simulink model "AirCtl_Mon"  (R2016b)
settings: configuration reference "CodeGenConfigSet" (kept outside this file)
values from neighbouring files (symbols this model uses):
  AirCtl_dnEngTrans_C = Calibration.Parameter    [init_AirCtl_Mon.m]    (also in init_AirCtl_Mon_SIL.m = Simulink.Parameter)
  AirCtl_dqLeadTrans_C = Calibration.Parameter    [init_AirCtl_Mon.m]    (also in init_AirCtl_Mon_SIL.m = Simulink.Parameter)
  AirCtl_drAPPTrans_C = Calibration.Parameter    [init_AirCtl_Mon.m]    (also in init_AirCtl_Mon_SIL.m = Simulink.Parameter)
  AirCtl_facActDesVal_C = Calibration.Parameter    [init_AirCtl_Mon.m]    (also in init_AirCtl_Mon_SIL.m = Simulink.Parameter)
  AirCtl_facEngTempSmkHysCor_CUR = Calibration.Parameter    [init_AirCtl_Mon.m]    (also in init_AirCtl_Mon_SIL.m = Simulink.Parameter)
  AirCtl_facEngTempSmkHysCor_CURX = Calibration.Parameter    [init_AirCtl_Mon.m]    (also in init_AirCtl_Mon_SIL.m = Simulink.Parameter)
  AirCtl_facEnvPresSmkHysCor_CUR = Calibration.Parameter    [init_AirCtl_Mon.m]    (also in init_AirCtl_Mon_SIL.m = Simulink.Parameter)
  AirCtl_facEnvPresSmkHysCor_CURX = Calibration.Parameter    [init_AirCtl_Mon.m]    (also in init_AirCtl_Mon_SIL.m = Simulink.Parameter)
  AirCtl_mMaxDvt_MAP = Calibration.Parameter    [init_AirCtl_Mon.m]    (also in init_AirCtl_Mon_SIL.m = Simulink.Parameter)
  AirCtl_mMaxDvt_MAPX = Calibration.Parameter    [init_AirCtl_Mon.m]    (also in init_AirCtl_Mon_SIL.m = Simulink.Parameter)
  AirCtl_mMaxDvt_MAPY = Calibration.Parameter    [init_AirCtl_Mon.m]    (also in init_AirCtl_Mon_SIL.m = Simulink.Parameter)
  AirCtl_mMinDvt_MAP = Calibration.Parameter    [init_AirCtl_Mon.m]    (also in init_AirCtl_Mon_SIL.m = Simulink.Parameter)
  AirCtl_mMinDvt_MAPX = Calibration.Parameter    [init_AirCtl_Mon.m]    (also in init_AirCtl_Mon_SIL.m = Simulink.Parameter)
  AirCtl_mMinDvt_MAPY = Calibration.Parameter    [init_AirCtl_Mon.m]    (also in init_AirCtl_Mon_SIL.m = Simulink.Parameter)
  AirCtl_nLoIdl_C = Calibration.Parameter    [init_AirCtl_Mon.m]    (also in init_AirCtl_Mon_SIL.m = Simulink.Parameter)
  AirCtl_nOvrRun_C = Calibration.Parameter    [init_AirCtl_Mon.m]    (also in init_AirCtl_Mon_SIL.m = Simulink.Parameter)
  AirCtl_numAirTempMon_C = Calibration.Parameter    [init_AirCtl_Mon.m]    (also in init_AirCtl_Mon_SIL.m = Simulink.Parameter)
  AirCtl_numEngTempMon_C = Calibration.Parameter    [init_AirCtl_Mon.m]    (also in init_AirCtl_Mon_SIL.m = Simulink.Parameter)
  AirCtl_pAirHi_C = Calibration.Parameter    [init_AirCtl_Mon.m]    (also in init_AirCtl_Mon_SIL.m = Simulink.Parameter)
  AirCtl_pAirLo_C = Calibration.Parameter    [init_AirCtl_Mon.m]    (also in init_AirCtl_Mon_SIL.m = Simulink.Parameter)
  AirCtl_qEngTempSmkHysCor_MAP = Calibration.Parameter    [init_AirCtl_Mon.m]    (also in init_AirCtl_Mon_SIL.m = Simulink.Parameter)
  AirCtl_qEngTempSmkHysCor_MAPX = Calibration.Parameter    [init_AirCtl_Mon.m]    (also in init_AirCtl_Mon_SIL.m = Simulink.Parameter)
  AirCtl_qEngTempSmkHysCor_MAPY = Calibration.Parameter    [init_AirCtl_Mon.m]    (also in init_AirCtl_Mon_SIL.m = Simulink.Parameter)
  AirCtl_qEnvPresSmkHysCor_MAP = Calibration.Parameter    [init_AirCtl_Mon.m]    (also in init_AirCtl_Mon_SIL.m = Simulink.Parameter)
  AirCtl_qEnvPresSmkHysCor_MAPX = Calibration.Parameter    [init_AirCtl_Mon.m]    (also in init_AirCtl_Mon_SIL.m = Simulink.Parameter)
  AirCtl_qEnvPresSmkHysCor_MAPY = Calibration.Parameter    [init_AirCtl_Mon.m]    (also in init_AirCtl_Mon_SIL.m = Simulink.Parameter)
  AirCtl_qOvrRun_C = Calibration.Parameter    [init_AirCtl_Mon.m]    (also in init_AirCtl_Mon_SIL.m = Simulink.Parameter)
  AirCtl_qSmkHys_MAP = Calibration.Parameter    [init_AirCtl_Mon.m]    (also in init_AirCtl_Mon_SIL.m = Simulink.Parameter)
  AirCtl_qSmkHys_MAPX = Calibration.Parameter    [init_AirCtl_Mon.m]    (also in init_AirCtl_Mon_SIL.m = Simulink.Parameter)
  AirCtl_qSmkHys_MAPY = Calibration.Parameter    [init_AirCtl_Mon.m]    (also in init_AirCtl_Mon_SIL.m = Simulink.Parameter)
  AirCtl_qSwtSmkHi_C = Calibration.Parameter    [init_AirCtl_Mon.m]    (also in init_AirCtl_Mon_SIL.m = Simulink.Parameter)
  AirCtl_qSwtSmkLo_C = Calibration.Parameter    [init_AirCtl_Mon.m]    (also in init_AirCtl_Mon_SIL.m = Simulink.Parameter)
  AirCtl_rEGRDflVal_CA = Calibration.Parameter    [init_AirCtl_Mon.m]    (also in init_AirCtl_Mon_SIL.m = Simulink.Parameter)
  AirCtl_rTVADflVal_CA = Calibration.Parameter    [init_AirCtl_Mon.m]    (also in init_AirCtl_Mon_SIL.m = Simulink.Parameter)
  AirCtl_stPrioMon_CA = Calibration.Parameter    [init_AirCtl_Mon.m]    (also in init_AirCtl_Mon_SIL.m = Simulink.Parameter)
  AirCtl_swtGovDvtMonEna_C = Calibration.Parameter    [init_AirCtl_Mon.m]    (also in init_AirCtl_Mon_SIL.m = Simulink.Parameter)
  AirCtl_tAirCldHi_C = Calibration.Parameter    [init_AirCtl_Mon.m]    (also in init_AirCtl_Mon_SIL.m = Simulink.Parameter)
  AirCtl_tAirCldLo_C = Calibration.Parameter    [init_AirCtl_Mon.m]    (also in init_AirCtl_Mon_SIL.m = Simulink.Parameter)
  AirCtl_tAirWrmHi_C = Calibration.Parameter    [init_AirCtl_Mon.m]    (also in init_AirCtl_Mon_SIL.m = Simulink.Parameter)
  AirCtl_tAirWrmLo_C = Calibration.Parameter    [init_AirCtl_Mon.m]    (also in init_AirCtl_Mon_SIL.m = Simulink.Parameter)
  AirCtl_tClntCldHi_C = Calibration.Parameter    [init_AirCtl_Mon.m]    (also in init_AirCtl_Mon_SIL.m = Simulink.Parameter)
  AirCtl_tClntCldLo_C = Calibration.Parameter    [init_AirCtl_Mon.m]    (also in init_AirCtl_Mon_SIL.m = Simulink.Parameter)
  AirCtl_tClntWrmHi_C = Calibration.Parameter    [init_AirCtl_Mon.m]    (also in init_AirCtl_Mon_SIL.m = Simulink.Parameter)
  AirCtl_tClntWrmLo_C = Calibration.Parameter    [init_AirCtl_Mon.m]    (also in init_AirCtl_Mon_SIL.m = Simulink.Parameter)
  AirCtl_tiCldStrt_CUR = Calibration.Parameter    [init_AirCtl_Mon.m]    (also in init_AirCtl_Mon_SIL.m = Simulink.Parameter)
  AirCtl_tiCldStrt_CURX = Calibration.Parameter    [init_AirCtl_Mon.m]    (also in init_AirCtl_Mon_SIL.m = Simulink.Parameter)
  AirCtl_tiClth_C = Calibration.Parameter    [init_AirCtl_Mon.m]    (also in init_AirCtl_Mon_SIL.m = Simulink.Parameter)
  AirCtl_tiDynSmkDly_C = Calibration.Parameter    [init_AirCtl_Mon.m]    (also in init_AirCtl_Mon_SIL.m = Simulink.Parameter)
  AirCtl_tiGovDvtMaxDebDef_C = Calibration.Parameter    [init_AirCtl_Mon.m]    (also in init_AirCtl_Mon_SIL.m = Simulink.Parameter)
  AirCtl_tiGovDvtMaxDebOk_C = Calibration.Parameter    [init_AirCtl_Mon.m]    (also in init_AirCtl_Mon_SIL.m = Simulink.Parameter)
  AirCtl_tiGovDvtMinDebDef_C = Calibration.Parameter    [init_AirCtl_Mon.m]    (also in init_AirCtl_Mon_SIL.m = Simulink.Parameter)
  AirCtl_tiGovDvtMinDebOk_C = Calibration.Parameter    [init_AirCtl_Mon.m]    (also in init_AirCtl_Mon_SIL.m = Simulink.Parameter)
  AirCtl_tiLoIdl_C = Calibration.Parameter    [init_AirCtl_Mon.m]    (also in init_AirCtl_Mon_SIL.m = Simulink.Parameter)
  AirCtl_tiStatSmkDly_C = Calibration.Parameter    [init_AirCtl_Mon.m]    (also in init_AirCtl_Mon_SIL.m = Simulink.Parameter)
  AirCtl_tiTransDly_C = Calibration.Parameter    [init_AirCtl_Mon.m]    (also in init_AirCtl_Mon_SIL.m = Simulink.Parameter)
  AirCtl_uBattThres_C = Calibration.Parameter    [init_AirCtl_Mon.m]    (also in init_AirCtl_Mon_SIL.m = Simulink.Parameter)
  ASMod_numBnk_C = Calibration.Parameter    [init_AirCtl_Mon.m]    (also in init_AirCtl_Mon_SIL.m = Simulink.Parameter)
  Epm_numCyl_C = Calibration.Parameter    [init_AirCtl_Mon.m]    (also in init_AirCtl_Mon_SIL.m = Simulink.Parameter)
undefined symbols (not defined in the file or in its folder): AirCtl_Mon_DT, EngState_conv, Switch_conv
libraries: simulink x45, CXLib x23
(part 2 of 4)

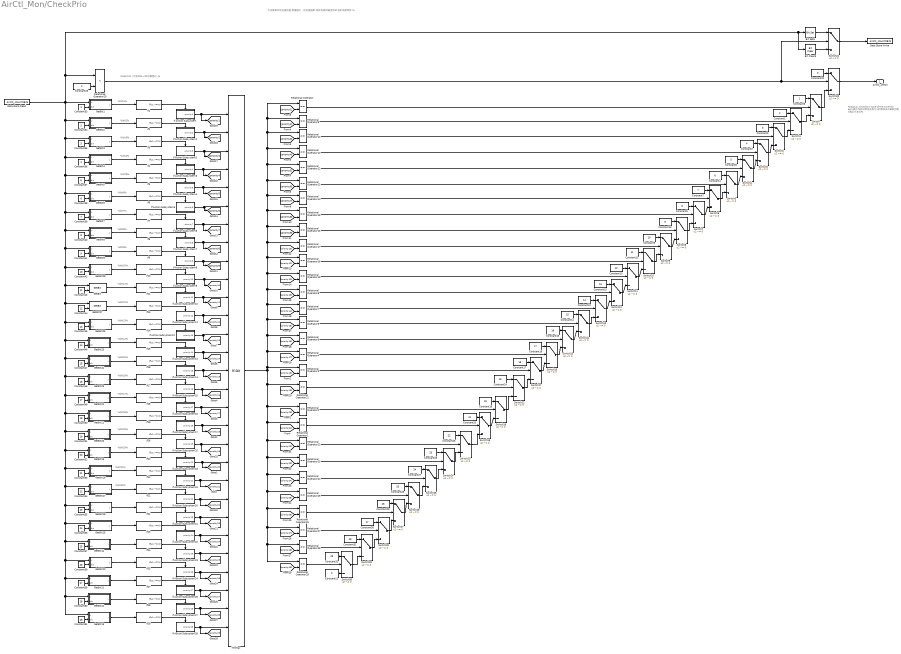
== system AirCtl_Mon/CheckPrio ==
  note: %bit19%
  note: %bit22%
  note: %bit21%
  note: %bit20%
  note: %bit18%
  note: %bit17%
  note: %bit16%
  note: %bit15%
  note: %bit14%
  note: %bit13%
  note: %bit12%
  note: %bit11%
  note: %bit10%
  note: %bit9%
  note: %bit8%
  note: %bit7%
  note: %bit6%
  note: %bit5%
  note: %bit4%
  note: %bit3%
  note: %关断条件优先级检查
      | 数值越大，优先级越高,同优先级时输出低bit位的关断条件 %
  note: %Status: shutdown case of the governor
      | eg:1表示当前中断优先级为1的请求关闭EGR控制
      | 0表示不关闭%
  note: %bit1%
  note: %bit2%
  note: %Normal（所有bit1~31位都是0）%
  Bit Clear5 : simulink/Logic and Bit Operations/Bit Clear  iBit=0
  Bit Set5 : simulink/Logic and Bit Operations/Bit Set  iBit=0
  Constant1 : Constant  Value=2  OutDataTypeStr=Inherit: Inherit via back propagation
  Constant10 : Constant  Value=12  OutDataTypeStr=Inherit: Inherit via back propagation
  Constant11 : Constant  Value=11  OutDataTypeStr=Inherit: Inherit via back propagation
  Constant12 : Constant  Value=14  OutDataTypeStr=Inherit: Inherit via back propagation
  Constant13 : Constant  Value=9  OutDataTypeStr=Inherit: Inherit via back propagation
  Constant14 : Constant  Value=15  OutDataTypeStr=Inherit: Inherit via back propagation
  Constant15 : Constant  Value=13  OutDataTypeStr=Inherit: Inherit via back propagation
  Constant16 : Constant  Value=16  OutDataTypeStr=Inherit: Inherit via back propagation
  Constant17 : Constant  Value=18  OutDataTypeStr=Inherit: Inherit via back propagation
  Constant18 : Constant  Value=20  OutDataTypeStr=Inherit: Inherit via back propagation
  Constant19 : Constant  Value=17  OutDataTypeStr=Inherit: Inherit via back propagation
  Constant2 : Constant  Value=4  OutDataTypeStr=Inherit: Inherit via back propagation
  Constant20 : Constant  Value=21  OutDataTypeStr=Inherit: Inherit via back propagation
  Constant21 : Constant  Value=0  OutDataTypeStr=Inherit: Inherit via back propagation
  Constant22 : Constant  Value=0  OutDataTypeStr=Inherit: Inherit via back propagation
  Constant23 : Constant  RequirementInfo={'other' 'APP_requirements.doc' '@Simulink_requirement_item_25' 'true' '手动开关' '' } %GIDa_9ff8e7a4_19db_42e9_b888_d3f27c0a2a42  Value=2  OutDataTypeStr=Inherit: Inherit via back propagation
  Constant24 : Constant  Value=19  OutDataTypeStr=Inherit: Inherit via back propagation
  Constant25 : Constant  Value=22  OutDataTypeStr=Inherit: Inherit via back propagation
  Constant26 : Constant  Value=23  OutDataTypeStr=Inherit: Inherit via back propagation
  Constant27 : Constant  Value=24  OutDataTypeStr=Inherit: Inherit via back propagation
  Constant28 : Constant  Value=25  OutDataTypeStr=Inherit: Inherit via back propagation
  Constant29 : Constant  Value=26  OutDataTypeStr=Inherit: Inherit via back propagation
  Constant3 : Constant  Value=3  OutDataTypeStr=Inherit: Inherit via back propagation
  Constant30 : Constant  Value=27  OutDataTypeStr=Inherit: Inherit via back propagation
  Constant31 : Constant  Value=28  OutDataTypeStr=Inherit: Inherit via back propagation
  Constant32 : Constant  Value=29  OutDataTypeStr=Inherit: Inherit via back propagation
  Constant33 : Constant  RequirementInfo={'other' 'APP_requirements.doc' '@Simulink_requirement_item_25' 'true' '手动开关' '' } %GIDa_8dd0c6e6_ea60_49d7_b46b_ab438e246230  OutDataTypeStr=uint8
  Constant34 : Constant  RequirementInfo={'other' 'APP_requirements.doc' '@Simulink_requirement_item_25' 'true' '手动开关' '' } %GIDa_459ecf2d_1b52_475d_81cc_86f88ae0e37a  Value=2  OutDataTypeStr=uint8
  Constant35 : Constant  RequirementInfo={'other' 'APP_requirements.doc' '@Simulink_requirement_item_25' 'true' '手动开关' '' } %GIDa_97e984dd_1262_4f1a_9e3f_0a8a4847e8c2  Value=3  OutDataTypeStr=uint8
  Constant36 : Constant  RequirementInfo={'other' 'APP_requirements.doc' '@Simulink_requirement_item_25' 'true' '手动开关' '' } %GIDa_aa429387_abff_4eca_a451_a653185f5261  Value=4  OutDataTypeStr=uint8
  Constant37 : Constant  RequirementInfo={'other' 'APP_requirements.doc' '@Simulink_requirement_item_25' 'true' '手动开关' '' } %GIDa_776b4e53_2600_48a2_98f3_ffb76672e236  Value=5  OutDataTypeStr=uint8
  Constant38 : Constant  RequirementInfo={'other' 'APP_requirements.doc' '@Simulink_requirement_item_25' 'true' '手动开关' '' } %GIDa_ddf4af35_e8ad_4358_ac5e_41e65ce97660  Value=6  OutDataTypeStr=uint8
  Constant39 : Constant  RequirementInfo={'other' 'APP_requirements.doc' '@Simulink_requirement_item_25' 'true' '手动开关' '' } %GIDa_3b276e3f_0951_4f1b_a061_4011452ae43f  Value=7  OutDataTypeStr=uint8
  Constant4 : Constant  Value=6  OutDataTypeStr=Inherit: Inherit via back propagation
  Constant40 : Constant  RequirementInfo={'other' 'APP_requirements.doc' '@Simulink_requirement_item_25' 'true' '手动开关' '' } %GIDa_b9eaab6f_8a8e_49ac_a677_53240963e0c3  Value=8  OutDataTypeStr=uint8
  Constant41 : Constant  RequirementInfo={'other' 'APP_requirements.doc' '@Simulink_requirement_item_25' 'true' '手动开关' '' } %GIDa_01aedbb6_55a6_4a21_a0ea_ad9cf4615d3d  Value=9  OutDataTypeStr=uint8
  Constant42 : Constant  RequirementInfo={'other' 'APP_requirements.doc' '@Simulink_requirement_item_25' 'true' '手动开关' '' } %GIDa_614a409c_4c3d_41e4_a7d0_053ba21c259b  Value=10  OutDataTypeStr=uint8
  Constant43 : Constant  RequirementInfo={'other' 'APP_requirements.doc' '@Simulink_requirement_item_25' 'true' '手动开关' '' } %GIDa_3c5ad0e3_a2b8_4859_a02a_30a23b08bfa3  Value=11  OutDataTypeStr=uint8
  Constant44 : Constant  RequirementInfo={'other' 'APP_requirements.doc' '@Simulink_requirement_item_25' 'true' '手动开关' '' } %GIDa_6f7af695_7339_4028_b949_7c524a37f015  Value=12  OutDataTypeStr=uint8
  Constant45 : Constant  RequirementInfo={'other' 'APP_requirements.doc' '@Simulink_requirement_item_25' 'true' '手动开关' '' } %GIDa_1ca5f349_8ebd_45d0_9976_f298523343d5  Value=13  OutDataTypeStr=uint8
  Constant46 : Constant  RequirementInfo={'other' 'APP_requirements.doc' '@Simulink_requirement_item_25' 'true' '手动开关' '' } %GIDa_45ac18be_7d7f_4385_bdfc_d66e5efb5d38  Value=14  OutDataTypeStr=uint8
  Constant47 : Constant  RequirementInfo={'other' 'APP_requirements.doc' '@Simulink_requirement_item_25' 'true' '手动开关' '' } %GIDa_1dc524ca_7018_4f76_b638_f454eb045857  Value=15  OutDataTypeStr=uint8
  Constant48 : Constant  RequirementInfo={'other' 'APP_requirements.doc' '@Simulink_requirement_item_25' 'true' '手动开关' '' } %GIDa_ae9f18e3_e472_4c5c_9282_7547ae504b7f  Value=16  OutDataTypeStr=uint8
  Constant49 : Constant  RequirementInfo={'other' 'APP_requirements.doc' '@Simulink_requirement_item_25' 'true' '手动开关' '' } %GIDa_b1ce1e54_f70c_4d0c_8eb8_07a2756ee938  Value=17  OutDataTypeStr=uint8
  Constant5 : Constant  Value=8  OutDataTypeStr=Inherit: Inherit via back propagation
  Constant50 : Constant  RequirementInfo={'other' 'APP_requirements.doc' '@Simulink_requirement_item_25' 'true' '手动开关' '' } %GIDa_303cbb98_88c5_4afc_ab22_77a2530af4c9  Value=18  OutDataTypeStr=uint8
  Constant51 : Constant  RequirementInfo={'other' 'APP_requirements.doc' '@Simulink_requirement_item_25' 'true' '手动开关' '' } %GIDa_cc84696b_14f0_4e97_853b_a4b589dd5f06  Value=19  OutDataTypeStr=uint8
  Constant52 : Constant  RequirementInfo={'other' 'APP_requirements.doc' '@Simulink_requirement_item_25' 'true' '手动开关' '' } %GIDa_43d761b0_2e5d_4aee_9c98_00f17b135858  Value=20  OutDataTypeStr=uint8
  Constant53 : Constant  RequirementInfo={'other' 'APP_requirements.doc' '@Simulink_requirement_item_25' 'true' '手动开关' '' } %GIDa_913b2337_2a88_4a1b_bba1_427d36531b8f  Value=21  OutDataTypeStr=uint8
  Constant54 : Constant  RequirementInfo={'other' 'APP_requirements.doc' '@Simulink_requirement_item_25' 'true' '手动开关' '' } %GIDa_a6ee6852_5445_447b_8cc3_6664092024ff  Value=22  OutDataTypeStr=uint8
  Constant55 : Constant  RequirementInfo={'other' 'APP_requirements.doc' '@Simulink_requirement_item_25' 'true' '手动开关' '' } %GIDa_c6d134ba_cb1f_4692_bcae_df29b739cc4f  Value=23  OutDataTypeStr=uint8
  Constant56 : Constant  RequirementInfo={'other' 'APP_requirements.doc' '@Simulink_requirement_item_25' 'true' '手动开关' '' } %GIDa_0ea449e8_8fde_4c16_a22d_50abb736ba60  Value=24  OutDataTypeStr=uint8
  Constant57 : Constant  RequirementInfo={'other' 'APP_requirements.doc' '@Simulink_requirement_item_25' 'true' '手动开关' '' } %GIDa_5643493f_e627_45e5_b17d_7ec49479d6fd  Value=25  OutDataTypeStr=uint8
  Constant58 : Constant  RequirementInfo={'other' 'APP_requirements.doc' '@Simulink_requirement_item_25' 'true' '手动开关' '' } %GIDa_fe056d5d_c71d_4fc7_ae76_b415e00f1938  Value=26  OutDataTypeStr=uint8
  Constant59 : Constant  RequirementInfo={'other' 'APP_requirements.doc' '@Simulink_requirement_item_25' 'true' '手动开关' '' } %GIDa_cfc02ad7_2f9a_4174_a8f4_b5e41cfc54dd  Value=27  OutDataTypeStr=uint8
  Constant6 : Constant  OutDataTypeStr=Inherit: Inherit via back propagation
  Constant60 : Constant  RequirementInfo={'other' 'APP_requirements.doc' '@Simulink_requirement_item_25' 'true' '手动开关' '' } %GIDa_0584c89f_78e3_40ae_ad7e_f84076556add  Value=28  OutDataTypeStr=uint8
  Constant61 : Constant  RequirementInfo={'other' 'APP_requirements.doc' '@Simulink_requirement_item_25' 'true' '手动开关' '' } %GIDa_3756beae_2b11_40ae_acb4_cf862cd3842f  Value=29  OutDataTypeStr=uint8
  Constant7 : Constant  Value=7  OutDataTypeStr=Inherit: Inherit via back propagation
  Constant8 : Constant  Value=5  OutDataTypeStr=Inherit: Inherit via back propagation
  Constant9 : Constant  Value=10  OutDataTypeStr=Inherit: Inherit via back propagation
  Data Store Read : DataStoreRead  DataStoreName=AirCtl_stAirCtlBits
  Data Store Write : DataStoreWrite  DataStoreName=AirCtl_stAirCtlBits
  GetBit : CXLib/GetBit  dataTypeString=uint32  dataLength=0
      settings: AttributesFormatString=Get bit from %<dataTypeString>
  GetBit1 : Subsystem  mask(GetBit){dataTypeString=uint32, dataLength=0}
      mask prompts: dataTypeString "Input Data Type"; dataLength "DataType Length"
      mask help:
      | Acquires the value of the bit specified by the position (zero indexed).
      |
      | Output is always boolean.
      |
      | INPUTS:
      | u - input value
      | bit - position of bit to get (uint8)
      |
      | OUTPUTS:
      | y - output value
      mask init:
      | %Initial data type length info.
      | switch dataTypeString
      |     case 'uint8'
      |         dataLength=8;
      |     case 'uint16'
      |         dataLength=16;
      |     case 'uint32'
      |         dataLength=32;
      |     otherwise
      |         error('Unexpected data type define!')
      | end
      | set_param([gcb,'/u'],'OutDataTypeStr',dataTypeString)
      settings: AttributesFormatString=Get bit from %<dataTypeString>
      mask Display: image(imread('GETBIT.jpg'),[0.2,0.2,0.6,0.6]);
  GetBit10 : Subsystem  mask(GetBit){dataTypeString=uint32, dataLength=0}
      mask prompts: dataTypeString "Input Data Type"; dataLength "DataType Length"
      mask help:
      | Acquires the value of the bit specified by the position (zero indexed).
      |
      | Output is always boolean.
      |
      | INPUTS:
      | u - input value
      | bit - position of bit to get (uint8)
      |
      | OUTPUTS:
      | y - output value
      mask init: same as AirCtl_Mon/CheckPrio/GetBit1
      settings: AttributesFormatString=Get bit from %<dataTypeString>
      mask Display: image(imread('GETBIT.jpg'),[0.2,0.2,0.6,0.6]);
  GetBit11 : Subsystem  mask(GetBit){dataTypeString=uint32, dataLength=0}
      mask prompts: dataTypeString "Input Data Type"; dataLength "DataType Length"
      mask help:
      | Acquires the value of the bit specified by the position (zero indexed).
      |
      | Output is always boolean.
      |
      | INPUTS:
      | u - input value
      | bit - position of bit to get (uint8)
      |
      | OUTPUTS:
      | y - output value
      mask init: same as AirCtl_Mon/CheckPrio/GetBit1
      settings: AttributesFormatString=Get bit from %<dataTypeString>
      mask Display: image(imread('GETBIT.jpg'),[0.2,0.2,0.6,0.6]);
  GetBit12 : Subsystem  mask(GetBit){dataTypeString=uint32, dataLength=0}
      mask prompts: dataTypeString "Input Data Type"; dataLength "DataType Length"
      mask help:
      | Acquires the value of the bit specified by the position (zero indexed).
      |
      | Output is always boolean.
      |
      | INPUTS:
      | u - input value
      | bit - position of bit to get (uint8)
      |
      | OUTPUTS:
      | y - output value
      mask init: same as AirCtl_Mon/CheckPrio/GetBit1
      settings: AttributesFormatString=Get bit from %<dataTypeString>
      mask Display: image(imread('GETBIT.jpg'),[0.2,0.2,0.6,0.6]);
  GetBit13 : Subsystem  mask(GetBit){dataTypeString=uint32, dataLength=0}
      mask prompts: dataTypeString "Input Data Type"; dataLength "DataType Length"
      mask help:
      | Acquires the value of the bit specified by the position (zero indexed).
      |
      | Output is always boolean.
      |
      | INPUTS:
      | u - input value
      | bit - position of bit to get (uint8)
      |
      | OUTPUTS:
      | y - output value
      mask init: same as AirCtl_Mon/CheckPrio/GetBit1
      settings: AttributesFormatString=Get bit from %<dataTypeString>
      mask Display: image(imread('GETBIT.jpg'),[0.2,0.2,0.6,0.6]);
  GetBit14 : Subsystem  mask(GetBit){dataTypeString=uint32, dataLength=0}
      mask prompts: dataTypeString "Input Data Type"; dataLength "DataType Length"
      mask help:
      | Acquires the value of the bit specified by the position (zero indexed).
      |
      | Output is always boolean.
      |
      | INPUTS:
      | u - input value
      | bit - position of bit to get (uint8)
      |
      | OUTPUTS:
      | y - output value
      mask init: same as AirCtl_Mon/CheckPrio/GetBit1
      settings: AttributesFormatString=Get bit from %<dataTypeString>
      mask Display: image(imread('GETBIT.jpg'),[0.2,0.2,0.6,0.6]);
  GetBit15 : Subsystem  mask(GetBit){dataTypeString=uint32, dataLength=0}
      mask prompts: dataTypeString "Input Data Type"; dataLength "DataType Length"
      mask help:
      | Acquires the value of the bit specified by the position (zero indexed).
      |
      | Output is always boolean.
      |
      | INPUTS:
      | u - input value
      | bit - position of bit to get (uint8)
      |
      | OUTPUTS:
      | y - output value
      mask init: same as AirCtl_Mon/CheckPrio/GetBit1
      settings: AttributesFormatString=Get bit from %<dataTypeString>
      mask Display: image(imread('GETBIT.jpg'),[0.2,0.2,0.6,0.6]);
  GetBit16 : Subsystem  mask(GetBit){dataTypeString=uint32, dataLength=0}
      mask prompts: dataTypeString "Input Data Type"; dataLength "DataType Length"
      mask help:
      | Acquires the value of the bit specified by the position (zero indexed).
      |
      | Output is always boolean.
      |
      | INPUTS:
      | u - input value
      | bit - position of bit to get (uint8)
      |
      | OUTPUTS:
      | y - output value
      mask init: same as AirCtl_Mon/CheckPrio/GetBit1
      settings: AttributesFormatString=Get bit from %<dataTypeString>
      mask Display: image(imread('GETBIT.jpg'),[0.2,0.2,0.6,0.6]);
  GetBit17 : Subsystem  mask(GetBit){dataTypeString=uint32, dataLength=0}
      mask prompts: dataTypeString "Input Data Type"; dataLength "DataType Length"
      mask help:
      | Acquires the value of the bit specified by the position (zero indexed).
      |
      | Output is always boolean.
      |
      | INPUTS:
      | u - input value
      | bit - position of bit to get (uint8)
      |
      | OUTPUTS:
      | y - output value
      mask init: same as AirCtl_Mon/CheckPrio/GetBit1
      settings: AttributesFormatString=Get bit from %<dataTypeString>
      mask Display: image(imread('GETBIT.jpg'),[0.2,0.2,0.6,0.6]);
  GetBit18 : Subsystem  mask(GetBit){dataTypeString=uint32, dataLength=0}
      mask prompts: dataTypeString "Input Data Type"; dataLength "DataType Length"
      mask help:
      | Acquires the value of the bit specified by the position (zero indexed).
      |
      | Output is always boolean.
      |
      | INPUTS:
      | u - input value
      | bit - position of bit to get (uint8)
      |
      | OUTPUTS:
      | y - output value
      mask init: same as AirCtl_Mon/CheckPrio/GetBit1
      settings: AttributesFormatString=Get bit from %<dataTypeString>
      mask Display: image(imread('GETBIT.jpg'),[0.2,0.2,0.6,0.6]);
  GetBit19 : Subsystem  mask(GetBit){dataTypeString=uint32, dataLength=0}
      mask prompts: dataTypeString "Input Data Type"; dataLength "DataType Length"
      mask help:
      | Acquires the value of the bit specified by the position (zero indexed).
      |
      | Output is always boolean.
      |
      | INPUTS:
      | u - input value
      | bit - position of bit to get (uint8)
      |
      | OUTPUTS:
      | y - output value
      mask init: same as AirCtl_Mon/CheckPrio/GetBit1
      settings: AttributesFormatString=Get bit from %<dataTypeString>
      mask Display: image(imread('GETBIT.jpg'),[0.2,0.2,0.6,0.6]);
  GetBit2 : Subsystem  mask(GetBit){dataTypeString=uint32, dataLength=0}
      mask prompts: dataTypeString "Input Data Type"; dataLength "DataType Length"
      mask help:
      | Acquires the value of the bit specified by the position (zero indexed).
      |
      | Output is always boolean.
      |
      | INPUTS:
      | u - input value
      | bit - position of bit to get (uint8)
      |
      | OUTPUTS:
      | y - output value
      mask init: same as AirCtl_Mon/CheckPrio/GetBit1
      settings: AttributesFormatString=Get bit from %<dataTypeString>
      mask Display: image(imread('GETBIT.jpg'),[0.2,0.2,0.6,0.6]);
  GetBit20 : Subsystem  mask(GetBit){dataTypeString=uint32, dataLength=0}
      mask prompts: dataTypeString "Input Data Type"; dataLength "DataType Length"
      mask help:
      | Acquires the value of the bit specified by the position (zero indexed).
      |
      | Output is always boolean.
      |
      | INPUTS:
      | u - input value
      | bit - position of bit to get (uint8)
      |
      | OUTPUTS:
      | y - output value
      mask init: same as AirCtl_Mon/CheckPrio/GetBit1
      settings: AttributesFormatString=Get bit from %<dataTypeString>
      mask Display: image(imread('GETBIT.jpg'),[0.2,0.2,0.6,0.6]);
  GetBit21 : Subsystem  mask(GetBit){dataTypeString=uint32, dataLength=0}
      mask prompts: dataTypeString "Input Data Type"; dataLength "DataType Length"
      mask help:
      | Acquires the value of the bit specified by the position (zero indexed).
      |
      | Output is always boolean.
      |
      | INPUTS:
      | u - input value
      | bit - position of bit to get (uint8)
      |
      | OUTPUTS:
      | y - output value
      mask init: same as AirCtl_Mon/CheckPrio/GetBit1
      settings: AttributesFormatString=Get bit from %<dataTypeString>
      mask Display: image(imread('GETBIT.jpg'),[0.2,0.2,0.6,0.6]);
  GetBit22 : Subsystem  mask(GetBit){dataTypeString=uint32, dataLength=0}
      mask prompts: dataTypeString "Input Data Type"; dataLength "DataType Length"
      mask help:
      | Acquires the value of the bit specified by the position (zero indexed).
      |
      | Output is always boolean.
      |
      | INPUTS:
      | u - input value
      | bit - position of bit to get (uint8)
      |
      | OUTPUTS:
      | y - output value
      mask init: same as AirCtl_Mon/CheckPrio/GetBit1
      settings: AttributesFormatString=Get bit from %<dataTypeString>
      mask Display: image(imread('GETBIT.jpg'),[0.2,0.2,0.6,0.6]);
  GetBit23 : Subsystem  mask(GetBit){dataTypeString=uint32, dataLength=0}
      mask prompts: dataTypeString "Input Data Type"; dataLength "DataType Length"
      mask help:
      | Acquires the value of the bit specified by the position (zero indexed).
      |
      | Output is always boolean.
      |
      | INPUTS:
      | u - input value
      | bit - position of bit to get (uint8)
      |
      | OUTPUTS:
      | y - output value
      mask init: same as AirCtl_Mon/CheckPrio/GetBit1
      settings: AttributesFormatString=Get bit from %<dataTypeString>
      mask Display: image(imread('GETBIT.jpg'),[0.2,0.2,0.6,0.6]);
  GetBit24 : Subsystem  mask(GetBit){dataTypeString=uint32, dataLength=0}
      mask prompts: dataTypeString "Input Data Type"; dataLength "DataType Length"
      mask help:
      | Acquires the value of the bit specified by the position (zero indexed).
      |
      | Output is always boolean.
      |
      | INPUTS:
      | u - input value
      | bit - position of bit to get (uint8)
      |
      | OUTPUTS:
      | y - output value
      mask init: same as AirCtl_Mon/CheckPrio/GetBit1
      settings: AttributesFormatString=Get bit from %<dataTypeString>
      mask Display: image(imread('GETBIT.jpg'),[0.2,0.2,0.6,0.6]);
  GetBit25 : Subsystem  mask(GetBit){dataTypeString=uint32, dataLength=0}
      mask prompts: dataTypeString "Input Data Type"; dataLength "DataType Length"
      mask help:
      | Acquires the value of the bit specified by the position (zero indexed).
      |
      | Output is always boolean.
      |
      | INPUTS:
      | u - input value
      | bit - position of bit to get (uint8)
      |
      | OUTPUTS:
      | y - output value
      mask init: same as AirCtl_Mon/CheckPrio/GetBit1
      settings: AttributesFormatString=Get bit from %<dataTypeString>
      mask Display: image(imread('GETBIT.jpg'),[0.2,0.2,0.6,0.6]);
  GetBit26 : Subsystem  mask(GetBit){dataTypeString=uint32, dataLength=0}
      mask prompts: dataTypeString "Input Data Type"; dataLength "DataType Length"
      mask help:
      | Acquires the value of the bit specified by the position (zero indexed).
      |
      | Output is always boolean.
      |
      | INPUTS:
      | u - input value
      | bit - position of bit to get (uint8)
      |
      | OUTPUTS:
      | y - output value
      mask init: same as AirCtl_Mon/CheckPrio/GetBit1
      settings: AttributesFormatString=Get bit from %<dataTypeString>
      mask Display: image(imread('GETBIT.jpg'),[0.2,0.2,0.6,0.6]);
  GetBit27 : CXLib/GetBit  dataTypeString=uint32  dataLength=0
      settings: AttributesFormatString=Get bit from %<dataTypeString>
  GetBit29 : Subsystem  mask(GetBit){dataTypeString=uint32, dataLength=0}
      mask prompts: dataTypeString "Input Data Type"; dataLength "DataType Length"
      mask help:
      | Acquires the value of the bit specified by the position (zero indexed).
      |
      | Output is always boolean.
      |
      | INPUTS:
      | u - input value
      | bit - position of bit to get (uint8)
      |
      | OUTPUTS:
      | y - output value
      mask init: same as AirCtl_Mon/CheckPrio/GetBit1
      settings: AttributesFormatString=Get bit from %<dataTypeString>
      mask Display: image(imread('GETBIT.jpg'),[0.2,0.2,0.6,0.6]);
  GetBit3 : Subsystem  mask(GetBit){dataTypeString=uint32, dataLength=0}
      mask prompts: dataTypeString "Input Data Type"; dataLength "DataType Length"
      mask help:
      | Acquires the value of the bit specified by the position (zero indexed).
      |
      | Output is always boolean.
      |
      | INPUTS:
      | u - input value
      | bit - position of bit to get (uint8)
      |
      | OUTPUTS:
      | y - output value
      mask init: same as AirCtl_Mon/CheckPrio/GetBit1
      settings: AttributesFormatString=Get bit from %<dataTypeString>
      mask Display: image(imread('GETBIT.jpg'),[0.2,0.2,0.6,0.6]);
  GetBit4 : Subsystem  mask(GetBit){dataTypeString=uint32, dataLength=0}
      mask prompts: dataTypeString "Input Data Type"; dataLength "DataType Length"
      mask help:
      | Acquires the value of the bit specified by the position (zero indexed).
      |
      | Output is always boolean.
      |
      | INPUTS:
      | u - input value
      | bit - position of bit to get (uint8)
      |
      | OUTPUTS:
      | y - output value
      mask init: same as AirCtl_Mon/CheckPrio/GetBit1
      settings: AttributesFormatString=Get bit from %<dataTypeString>
      mask Display: image(imread('GETBIT.jpg'),[0.2,0.2,0.6,0.6]);
  GetBit5 : Subsystem  mask(GetBit){dataTypeString=uint32, dataLength=0}
      mask prompts: dataTypeString "Input Data Type"; dataLength "DataType Length"
      mask help:
      | Acquires the value of the bit specified by the position (zero indexed).
      |
      | Output is always boolean.
      |
      | INPUTS:
      | u - input value
      | bit - position of bit to get (uint8)
      |
      | OUTPUTS:
      | y - output value
      mask init: same as AirCtl_Mon/CheckPrio/GetBit1
      settings: AttributesFormatString=Get bit from %<dataTypeString>
      mask Display: image(imread('GETBIT.jpg'),[0.2,0.2,0.6,0.6]);
  GetBit6 : Subsystem  mask(GetBit){dataTypeString=uint32, dataLength=0}
      mask prompts: dataTypeString "Input Data Type"; dataLength "DataType Length"
      mask help:
      | Acquires the value of the bit specified by the position (zero indexed).
      |
      | Output is always boolean.
      |
      | INPUTS:
      | u - input value
      | bit - position of bit to get (uint8)
      |
      | OUTPUTS:
      | y - output value
      mask init: same as AirCtl_Mon/CheckPrio/GetBit1
      settings: AttributesFormatString=Get bit from %<dataTypeString>
      mask Display: image(imread('GETBIT.jpg'),[0.2,0.2,0.6,0.6]);
  GetBit7 : Subsystem  mask(GetBit){dataTypeString=uint32, dataLength=0}
      mask prompts: dataTypeString "Input Data Type"; dataLength "DataType Length"
      mask help:
      | Acquires the value of the bit specified by the position (zero indexed).
      |
      | Output is always boolean.
      |
      | INPUTS:
      | u - input value
      | bit - position of bit to get (uint8)
      |
      | OUTPUTS:
      | y - output value
      mask init: same as AirCtl_Mon/CheckPrio/GetBit1
      settings: AttributesFormatString=Get bit from %<dataTypeString>
      mask Display: image(imread('GETBIT.jpg'),[0.2,0.2,0.6,0.6]);
  GetBit8 : Subsystem  mask(GetBit){dataTypeString=uint32, dataLength=0}
      mask prompts: dataTypeString "Input Data Type"; dataLength "DataType Length"
      mask help:
      | Acquires the value of the bit specified by the position (zero indexed).
      |
      | Output is always boolean.
      |
      | INPUTS:
      | u - input value
      | bit - position of bit to get (uint8)
      |
      | OUTPUTS:
      | y - output value
      mask init: same as AirCtl_Mon/CheckPrio/GetBit1
      settings: AttributesFormatString=Get bit from %<dataTypeString>
      mask Display: image(imread('GETBIT.jpg'),[0.2,0.2,0.6,0.6]);
  GetBit9 : Subsystem  mask(GetBit){dataTypeString=uint32, dataLength=0}
      mask prompts: dataTypeString "Input Data Type"; dataLength "DataType Length"
      mask help:
      | Acquires the value of the bit specified by the position (zero indexed).
      |
      | Output is always boolean.
      |
      | INPUTS:
      | u - input value
      | bit - position of bit to get (uint8)
      |
      | OUTPUTS:
      | y - output value
      mask init: same as AirCtl_Mon/CheckPrio/GetBit1
      settings: AttributesFormatString=Get bit from %<dataTypeString>
      mask Display: image(imread('GETBIT.jpg'),[0.2,0.2,0.6,0.6]);
  If Action Subsystem : Subsystem  TreatAsAtomicUnit=on
  If Action Subsystem1 : Subsystem  TreatAsAtomicUnit=on
  If Action Subsystem10 : Subsystem  TreatAsAtomicUnit=on
  If Action Subsystem11 : Subsystem  TreatAsAtomicUnit=on
  If Action Subsystem12 : Subsystem  TreatAsAtomicUnit=on
  If Action Subsystem13 : Subsystem  TreatAsAtomicUnit=on
  If Action Subsystem14 : Subsystem  TreatAsAtomicUnit=on
  If Action Subsystem15 : Subsystem  TreatAsAtomicUnit=on
  If Action Subsystem16 : Subsystem  TreatAsAtomicUnit=on
  If Action Subsystem17 : Subsystem  TreatAsAtomicUnit=on
  If Action Subsystem18 : Subsystem  TreatAsAtomicUnit=on
  If Action Subsystem19 : Subsystem  TreatAsAtomicUnit=on
  If Action Subsystem2 : Subsystem  TreatAsAtomicUnit=on
  If Action Subsystem20 : Subsystem  TreatAsAtomicUnit=on
  If Action Subsystem21 : Subsystem  TreatAsAtomicUnit=on
  If Action Subsystem22 : Subsystem  TreatAsAtomicUnit=on
  If Action Subsystem23 : Subsystem  TreatAsAtomicUnit=on
  If Action Subsystem24 : Subsystem  TreatAsAtomicUnit=on
  If Action Subsystem25 : Subsystem  TreatAsAtomicUnit=on
  If Action Subsystem26 : Subsystem  TreatAsAtomicUnit=on
  If Action Subsystem27 : Subsystem  TreatAsAtomicUnit=on
  If Action Subsystem28 : Subsystem  TreatAsAtomicUnit=on
  If Action Subsystem3 : Subsystem  TreatAsAtomicUnit=on
  If Action Subsystem4 : Subsystem  TreatAsAtomicUnit=on
  If Action Subsystem5 : Subsystem  TreatAsAtomicUnit=on
  If Action Subsystem6 : Subsystem  TreatAsAtomicUnit=on
  If Action Subsystem7 : Subsystem  TreatAsAtomicUnit=on
  If Action Subsystem8 : Subsystem  TreatAsAtomicUnit=on
  If Action Subsystem9 : Subsystem  TreatAsAtomicUnit=on
  If{1..29} (29 alike) : If  IfExpression=u1 ~= 0  ShowElse=off
  MinMax : MinMax  Function=max  Inputs=29  SaturateOnIntegerOverflow=on  InputSameDT=on
  Relational Operator{,1..19,21..29} (29 alike) : RelationalOperator  Operator===  OutDataTypeStr=boolean  RndMeth=Simplest  InputSameDT=on
  Relational Operator20 : RelationalOperator  Operator=<  OutDataTypeStr=boolean  RndMeth=Simplest  InputSameDT=on
  Switch{,1..30} (31 alike) : Switch  Criteria=u2 ~= 0  InputSameDT=on
  AirCtl_stMon : Outport
  wires:
  Constant21/1 -> Switch30/3
  [priority29] -> Relational Operator29/2
  Constant32/1 -> Switch30/1
  Switch30/1 -> Switch29/3
  Relational Operator29/1 -> Switch30/2
  Constant31/1 -> Switch29/1
  Switch29/1 -> Switch28/3
  Relational Operator28/1 -> Switch29/2
  [priority28] -> Relational Operator28/2
  Constant30/1 -> Switch28/1
  Switch28/1 -> Switch27/3
  Relational Operator27/1 -> Switch28/2
  [priority27] -> Relational Operator27/2
  Constant29/1 -> Switch27/1
  Relational Operator26/1 -> Switch27/2
  Switch27/1 -> Switch26/3
  [priority26] -> Relational Operator26/2
  Constant28/1 -> Switch26/1
  Switch26/1 -> Switch25/3
  Relational Operator25/1 -> Switch26/2
  [priority25] -> Relational Operator25/2
  Constant27/1 -> Switch25/1
  Switch25/1 -> Switch24/3
  Relational Operator24/1 -> Switch25/2
  [priority24] -> Relational Operator24/2
  Constant26/1 -> Switch24/1
  Switch24/1 -> Switch23/3
  Relational Operator23/1 -> Switch24/2
  [priority23] -> Relational Operator23/2
  Constant25/1 -> Switch23/1
  Relational Operator22/1 -> Switch23/2
  [priority22] -> Relational Operator22/2
  Constant24/1 -> Switch22/1
  Relational Operator21/1 -> Switch22/2
  Switch22/1 -> Switch17/3
  [priority19] -> Relational Operator21/2
  If Action Subsystem28/1(priority29) -> [priority29], MinMax/29
  If29/1 -> If Action Subsystem28/Action
  If Action Subsystem27/1(priority28) -> [priority28], MinMax/28
  If28/1 -> If Action Subsystem27/Action
  If Action Subsystem26/1(priority27) -> [priority27], MinMax/27
  If27/1 -> If Action Subsystem26/Action
  If Action Subsystem25/1(priority19) -> MinMax/19, [priority19]
  GetBit20/1(y) -> If26/1
  If26/1 -> If Action Subsystem25/Action
  If Action Subsystem20/1(priority22) -> [priority22], MinMax/22
  If Action Subsystem23/1(priority25) -> [priority25], MinMax/25
  If Action Subsystem18/1(priority20) -> [priority20], MinMax/20
  If Action Subsystem17/1(priority18) -> [priority18], MinMax/18
  If Action Subsystem19/1(priority21) -> [priority21], MinMax/21
  If Action Subsystem21/1(priority23) -> [priority23], MinMax/23
  If Action Subsystem22/1(priority24) -> [priority24], MinMax/24
  If Action Subsystem24/1(priority26) -> [priority26], MinMax/26
  If25/1 -> If Action Subsystem24/Action
  GetBit14/1(y) -> If24/1
  If24/1 -> If Action Subsystem23/Action
  GetBit15/1(y) -> If23/1
  If23/1 -> If Action Subsystem22/Action
  GetBit16/1(y) -> If22/1
  If22/1 -> If Action Subsystem21/Action
  GetBit17/1(y) -> If21/1
  If21/1 -> If Action Subsystem20/Action
  Switch21/1 -> Data Store Write/1
  Bit Set5/1 -> Switch21/1
  Bit Clear5/1 -> Switch21/3
  Constant23/1 -> Relational Operator20/2
  If Action Subsystem/1(priority1) -> MinMax/1, [priority1]
  Relational Operator20/1 -> Switch20/2, Switch21/2
  Switch20/1 -> AirCtl_stMon/1
  Constant22/1 -> Switch20/1
  MinMax/1 -> Relational Operator1/1, Relational Operator22/1, Relational Operator29/1, Relational Operator28/1, Relational Operator27/1, Relational Operator26/1, Relational Operator25/1, Relational Operator24/1, Relational Operator23/1, Relational Operator2/1, Relational Operator21/1, Relational Operator3/1, Relational Operator4/1, Relational Operator5/1, Relational Operator6/1, Relational Operator7/1, Relational Operator8/1, Relational Operator19/1, Relational Operator/1, Relational Operator9/1, Relational Operator10/1, Relational Operator11/1, Relational Operator12/1, Relational Operator13/1, Relational Operator14/1, Relational Operator15/1, Relational Operator16/1, Relational Operator17/1, Relational Operator18/1
  [priority17] -> Relational Operator4/2
  [priority16] -> Relational Operator5/2
  [priority15] -> Relational Operator6/2
  [priority14] -> Relational Operator7/2
  [priority13] -> Relational Operator8/2
  [priority12] -> Relational Operator19/2
  [priority11] -> Relational Operator18/2
  [priority10] -> Relational Operator17/2
  [priority9] -> Relational Operator16/2
  [priority8] -> Relational Operator15/2
  [priority7] -> Relational Operator14/2
  [priority6] -> Relational Operator13/2
  [priority5] -> Relational Operator12/2
  [priority4] -> Relational Operator11/2
  [priority3] -> Relational Operator10/2
  [priority2] -> Relational Operator9/2
  [priority1] -> Relational Operator/2
  [priority18] -> Relational Operator3/2
  Switch1/1 -> Switch/3
  [priority20] -> Relational Operator2/2
  [priority21] -> Relational Operator1/2
  Switch23/1 -> Switch19/3
  If Action Subsystem16/1(priority17) -> MinMax/17, [priority17]
  If Action Subsystem14/1(priority15) -> MinMax/15, [priority15]
  If Action Subsystem13/1(priority14) -> MinMax/14, [priority14]
  If Action Subsystem12/1(priority13) -> MinMax/13, [priority13]
  If Action Subsystem11/1(priority12) -> MinMax/12, [priority12]
  If Action Subsystem10/1(priority11) -> MinMax/11, [priority11]
  If Action Subsystem9/1(priority10) -> MinMax/10, [priority10]
  If Action Subsystem8/1(priority9) -> MinMax/9, [priority9]
  If Action Subsystem7/1(priority8) -> MinMax/8, [priority8]
  If Action Subsystem6/1(priority7) -> MinMax/7, [priority7]
  If Action Subsystem5/1(priority6) -> MinMax/6, [priority6]
  If Action Subsystem4/1(priority5) -> MinMax/5, [priority5]
  If Action Subsystem3/1(priority4) -> MinMax/4, [priority4]
  If Action Subsystem2/1(priority3) -> MinMax/3, [priority3]
  If Action Subsystem1/1(priority2) -> MinMax/2, [priority2]
  If Action Subsystem15/1(priority16) -> MinMax/16, [priority16]
  Switch16/1 -> Switch15/3
  Constant19/1 -> Switch16/1
  Relational Operator1/1 -> Switch19/2
  Relational Operator3/1 -> Switch17/2
  Switch18/1 -> Switch22/3
  Switch19/1 -> Switch18/3
  Constant20/1 -> Switch19/1
  Constant18/1 -> Switch18/1
  Relational Operator2/1 -> Switch18/2
  Switch17/1 -> Switch16/3
  Constant17/1 -> Switch17/1
  Relational Operator4/1 -> Switch16/2
  Switch8/1 -> Switch7/3
  Constant15/1 -> Switch12/1
  Switch12/1 -> Switch11/3
  Relational Operator5/1 -> Switch15/2
  Relational Operator7/1 -> Switch13/2
  Switch14/1 -> Switch13/3
  Switch15/1 -> Switch14/3
  Constant16/1 -> Switch15/1
  Constant14/1 -> Switch14/1
  Relational Operator6/1 -> Switch14/2
  Switch13/1 -> Switch12/3
  Constant12/1 -> Switch13/1
  Relational Operator8/1 -> Switch12/2
  Relational Operator19/1 -> Switch11/2
  Relational Operator17/1 -> Switch9/2
  Switch10/1 -> Switch9/3
  Switch11/1 -> Switch10/3
  Constant10/1 -> Switch11/1
  Constant11/1 -> Switch10/1
  Relational Operator18/1 -> Switch10/2
  Switch9/1 -> Switch8/3
  Constant9/1 -> Switch9/1
  Constant13/1 -> Switch8/1
  Relational Operator16/1 -> Switch8/2
  Constant8/1 -> Switch4/1
  Switch4/1 -> Switch3/3
  Relational Operator15/1 -> Switch7/2
  Relational Operator13/1 -> Switch5/2
  Switch6/1 -> Switch5/3
  Switch7/1 -> Switch6/3
  Constant5/1 -> Switch7/1
  Constant7/1 -> Switch6/1
  Relational Operator14/1 -> Switch6/2
  Switch5/1 -> Switch4/3
  Constant4/1 -> Switch5/1
  Relational Operator12/1 -> Switch4/2
  Relational Operator11/1 -> Switch3/2
  Relational Operator9/1 -> Switch1/2
  Switch2/1 -> Switch1/3
  Switch3/1 -> Switch2/3
  Constant2/1 -> Switch3/1
  Constant3/1 -> Switch2/1
  Relational Operator10/1 -> Switch2/2
  Constant1/1 -> Switch1/1
  Constant6/1 -> Switch/1
  Switch/1 -> Switch20/3
  Relational Operator/1 -> Switch/2
  GetBit18/1(y) -> If12/1
  GetBit19/1(y) -> If20/1
  GetBit21/1(y) -> If19/1
  GetBit22/1(y) -> If18/1
  GetBit23/1(y) -> If17/1
  GetBit25/1(y) -> If15/1
  GetBit26/1(y) -> If14/1
  GetBit27/1 -> If13/1
  GetBit/1 -> If11/1
  GetBit29/1(y) -> If10/1
  If12/1 -> If Action Subsystem19/Action
  If20/1 -> If Action Subsystem18/Action
  If19/1 -> If Action Subsystem17/Action
  If18/1 -> If Action Subsystem16/Action
  If17/1 -> If Action Subsystem15/Action
  If16/1 -> If Action Subsystem14/Action
  If15/1 -> If Action Subsystem13/Action
  If14/1 -> If Action Subsystem12/Action
  If13/1 -> If Action Subsystem11/Action
  If11/1 -> If Action Subsystem10/Action
  If10/1 -> If Action Subsystem9/Action
  If9/1 -> If Action Subsystem8/Action
  If8/1 -> If Action Subsystem7/Action
  If7/1 -> If Action Subsystem6/Action
  If6/1 -> If Action Subsystem5/Action
  If5/1 -> If Action Subsystem4/Action
  If4/1 -> If Action Subsystem3/Action
  If2/1 -> If Action Subsystem1/Action
  If1/1 -> If Action Subsystem/Action
  Constant33/1 -> GetBit1/2(bit)
  Constant34/1 -> GetBit2/2(bit)
  Constant35/1 -> GetBit3/2(bit)
  Constant36/1 -> GetBit4/2(bit)
  Constant37/1 -> GetBit5/2(bit)
  Constant38/1 -> GetBit6/2(bit)
  Constant39/1 -> GetBit7/2(bit)
  Constant40/1 -> GetBit8/2(bit)
  Constant41/1 -> GetBit9/2(bit)
  Constant42/1 -> GetBit29/2(bit)
  Constant43/1 -> GetBit/2
  Constant44/1 -> GetBit27/2
  Constant45/1 -> GetBit26/2(bit)
  Constant46/1 -> GetBit25/2(bit)
  Constant47/1 -> GetBit24/2(bit)
  Constant48/1 -> GetBit23/2(bit)
  Constant49/1 -> GetBit22/2(bit)
  Constant50/1 -> GetBit21/2(bit)
  Constant51/1 -> GetBit20/2(bit)
  Constant52/1 -> GetBit19/2(bit)
  Constant53/1 -> GetBit18/2(bit)
  Constant54/1 -> GetBit17/2(bit)
  Constant55/1 -> GetBit16/2(bit)
  Constant56/1 -> GetBit15/2(bit)
  Constant57/1 -> GetBit14/2(bit)
  Constant58/1 -> GetBit10/2(bit)
  Constant59/1 -> GetBit11/2(bit)
  Constant60/1 -> GetBit12/2(bit)
  Constant61/1 -> GetBit13/2(bit)
  Data Store Read/1 -> GetBit1/1(u), GetBit2/1(u), GetBit3/1(u), GetBit4/1(u), GetBit5/1(u), GetBit6/1(u), GetBit7/1(u), GetBit8/1(u), GetBit9/1(u), GetBit29/1(u), GetBit/1, GetBit27/1, GetBit26/1(u), GetBit25/1(u), GetBit24/1(u), GetBit23/1(u), GetBit22/1(u), GetBit21/1(u), GetBit20/1(u), GetBit19/1(u), GetBit18/1(u), GetBit17/1(u), GetBit16/1(u), GetBit15/1(u), GetBit14/1(u), GetBit10/1(u), GetBit11/1(u), GetBit13/1(u), GetBit12/1(u), Bit Set5/1, Bit Clear5/1, Relational Operator20/1
  If3/1 -> If Action Subsystem2/Action
  GetBit1/1(y) -> If1/1
  GetBit2/1(y) -> If2/1
  GetBit3/1(y) -> If3/1
  GetBit4/1(y) -> If4/1
  GetBit5/1(y) -> If5/1
  GetBit6/1(y) -> If6/1
  GetBit7/1(y) -> If7/1
  GetBit8/1(y) -> If8/1
  GetBit9/1(y) -> If9/1
  GetBit10/1(y) -> If25/1
  GetBit11/1(y) -> If27/1
  GetBit12/1(y) -> If28/1
  GetBit13/1(y) -> If29/1
  GetBit24/1(y) -> If16/1

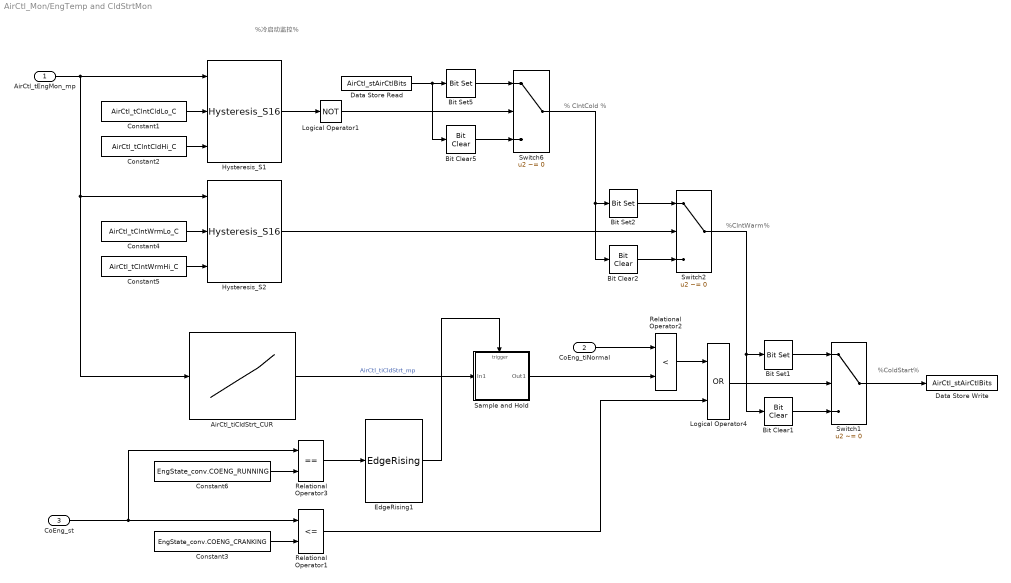
== system AirCtl_Mon/EngTemp and CldStrtMon ==
  note: %ClntWarm%
  note: %ColdStart%
  note: % ClntCold %
  note: %冷启动监控%
  AirCtl_tEngMon_mp : Inport
  CoEng_tiNormal : Inport  Port=2
  CoEng_st : Inport  Port=3
  AirCtl_tiCldStrt_CUR : Lookup_n-D  NumberOfTableDimensions=1  BreakpointsForDimension1=AirCtl_tiCldStrt_CURX  BeginIndexSearchUsingPreviousIndexResult=on  Table=AirCtl_tiCldStrt_CUR  TableDataTypeStr=Inherit: Inherit from 'Table data'  ExtrapMethod=Clip  UseLastTableValue=on  InternalRulePriority=Speed  OutDataTypeStr=Inherit: Inherit from 'Table data'  RndMeth=Simplest  SaturateOnIntegerOverflow=on
  Bit Clear1 : simulink/Logic and Bit Operations/Bit Clear  iBit=17
  Bit Clear2 : simulink/Logic and Bit Operations/Bit Clear  iBit=16
  Bit Clear5 : simulink/Logic and Bit Operations/Bit Clear  iBit=15
  Bit Set1 : simulink/Logic and Bit Operations/Bit Set  iBit=17
  Bit Set2 : simulink/Logic and Bit Operations/Bit Set  iBit=16
  Bit Set5 : simulink/Logic and Bit Operations/Bit Set  iBit=15
  Constant1 : Constant  Value=AirCtl_tClntCldLo_C
  Constant2 : Constant  Value=AirCtl_tClntCldHi_C
  Constant3 : Constant  Value=EngState_conv.COENG_CRANKING  OutDataTypeStr=Inherit: Inherit via back propagation
  Constant4 : Constant  Value=AirCtl_tClntWrmLo_C
  Constant5 : Constant  Value=AirCtl_tClntWrmHi_C
  Constant6 : Constant  Value=EngState_conv.COENG_RUNNING  OutDataTypeStr=Inherit: Inherit via back propagation
  Data Store Read : DataStoreRead  DataStoreName=AirCtl_stAirCtlBits
  Data Store Write : DataStoreWrite  DataStoreName=AirCtl_stAirCtlBits
  EdgeRising1 : CXLib/EdgeRising
  Hysteresis_S1 : CXLib/Hysteresis_S16
  Hysteresis_S2 : CXLib/Hysteresis_S16
  Logical Operator1 : Logic  Operator=NOT  AllPortsSameDT=off  OutDataTypeStr=boolean
  Logical Operator4 : Logic  Operator=OR  OutDataTypeStr=boolean
  Relational Operator1 : RelationalOperator  Operator=<=  OutDataTypeStr=boolean  RndMeth=Simplest  InputSameDT=on
  Relational Operator2 : RelationalOperator  Operator=<  OutDataTypeStr=boolean  RndMeth=Simplest  InputSameDT=on
  Relational Operator3 : RelationalOperator  Operator===  OutDataTypeStr=boolean  RndMeth=Simplest  InputSameDT=on
  Sample and Hold : Subsystem
  Switch1 : Switch  Criteria=u2 ~= 0  SaturateOnIntegerOverflow=on  InputSameDT=on
  Switch2 : Switch  Criteria=u2 ~= 0  SaturateOnIntegerOverflow=on  InputSameDT=on
  Switch6 : Switch  Criteria=u2 ~= 0  SaturateOnIntegerOverflow=on  InputSameDT=on
  wires:
  AirCtl_tEngMon_mp/1 -> Hysteresis_S1/1, Hysteresis_S2/1, AirCtl_tiCldStrt_CUR/1
  AirCtl_tiCldStrt_CUR/1 -> Sample and Hold/1(In1)  "AirCtl_tiCldStrt_mp"
  Switch6/1 -> Bit Clear2/1, Bit Set2/1
  Switch2/1 -> Bit Clear1/1, Bit Set1/1
  Bit Clear2/1 -> Switch2/3
  Bit Set2/1 -> Switch2/1
  Constant5/1 -> Hysteresis_S2/3
  Constant4/1 -> Hysteresis_S2/2
  Switch1/1 -> Data Store Write/1
  Bit Clear1/1 -> Switch1/3
  Bit Set1/1 -> Switch1/1
  Logical Operator4/1 -> Switch1/2
  Data Store Read/1 -> Bit Set5/1, Bit Clear5/1
  Bit Clear5/1 -> Switch6/3
  Bit Set5/1 -> Switch6/1
  Logical Operator1/1 -> Switch6/2
  CoEng_tiNormal/1 -> Relational Operator2/1
  Relational Operator2/1 -> Logical Operator4/1
  Relational Operator1/1 -> Logical Operator4/2
  Relational Operator3/1 -> EdgeRising1/1
  CoEng_st/1 -> Relational Operator3/1, Relational Operator1/1
  Constant3/1 -> Relational Operator1/2
  Constant2/1 -> Hysteresis_S1/3
  Constant1/1 -> Hysteresis_S1/2
  Constant6/1 -> Relational Operator3/2
  Sample and Hold/1(Out1) -> Relational Operator2/2
  EdgeRising1/1 -> Sample and Hold/Trigger
  Hysteresis_S2/1 -> Switch2/2
  Hysteresis_S1/1 -> Logical Operator1/1

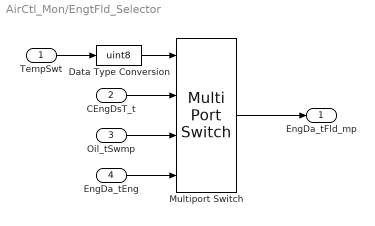
== system AirCtl_Mon/EngtFld_Selector ==
  TempSwt : Inport
  CEngDsT_t : Inport  Tag=deg  Description=engine coolant temperature after filter  Port=2
  Oil_tSwmp : Inport  Tag=deg  Description=Oil temperature in oil sump  Port=3
  EngDa_tEng : Inport  Tag=deg  Description=Engine temperature  Port=4
  Data Type Conversion : DataTypeConversion  OutDataTypeStr=uint8
  Multiport Switch : MultiPortSwitch  DataPortOrder=Zero-based contiguous
  EngDa_tFld_mp : Outport  Tag=deg  Description=Engine temperature field
  wires:
  CEngDsT_t/1 -> Multiport Switch/2
  Multiport Switch/1 -> EngDa_tFld_mp/1
  EngDa_tEng/1 -> Multiport Switch/4
  Oil_tSwmp/1 -> Multiport Switch/3
  Data Type Conversion/1 -> Multiport Switch/1
  TempSwt/1 -> Data Type Conversion/1
